simulink model "simple_controll"  (R2015b)
settings: Solver=FixedStepAuto  StartTime=0  StopTime=10  FixedStep=10*(1e-4)  RelTol=1e-3
undefined symbols (not defined in the file or in its folder): qc
libraries: simulink x4
settings Model: Creator=acsl  LastModifiedBy=acsl

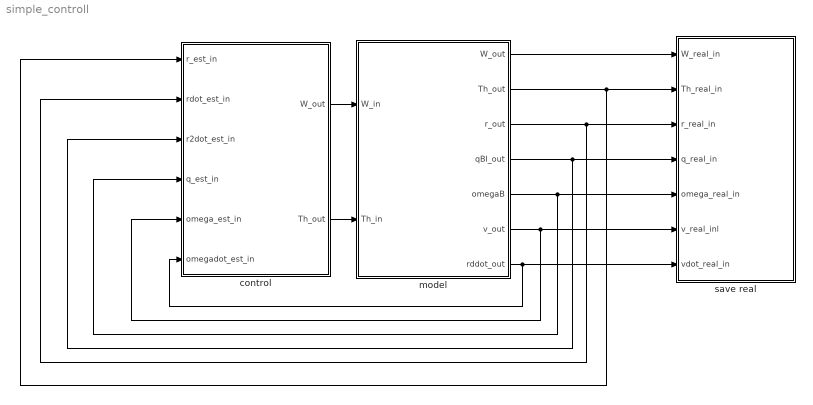
== system simple_controll ==
  control : Subsystem  InitFcn=init
  model : Subsystem
  save real : Subsystem
  wires:
  control/1(W_out) -> model/1(W_in)
  control/2(Th_out) -> model/2(Th_in)
  model/1(W_out) -> save real/1(W_real_in)
  model/2(Th_out) -> save real/2(Th_real_in), control/1(r_est_in)
  model/5(omegaB) -> save real/5(omega_real_in), control/4(q_est_in)
  model/6(v_out) -> save real/6(v_real_inl), control/5(omega_est_in)
  model/7(rddot_out) -> control/6(omegadot_est_in), save real/7(vdot_real_in)
  model/3(r_out) -> control/2(rdot_est_in), save real/3(r_real_in)
  model/4(qBI_out) -> save real/4(q_real_in), control/3(r2dot_est_in)

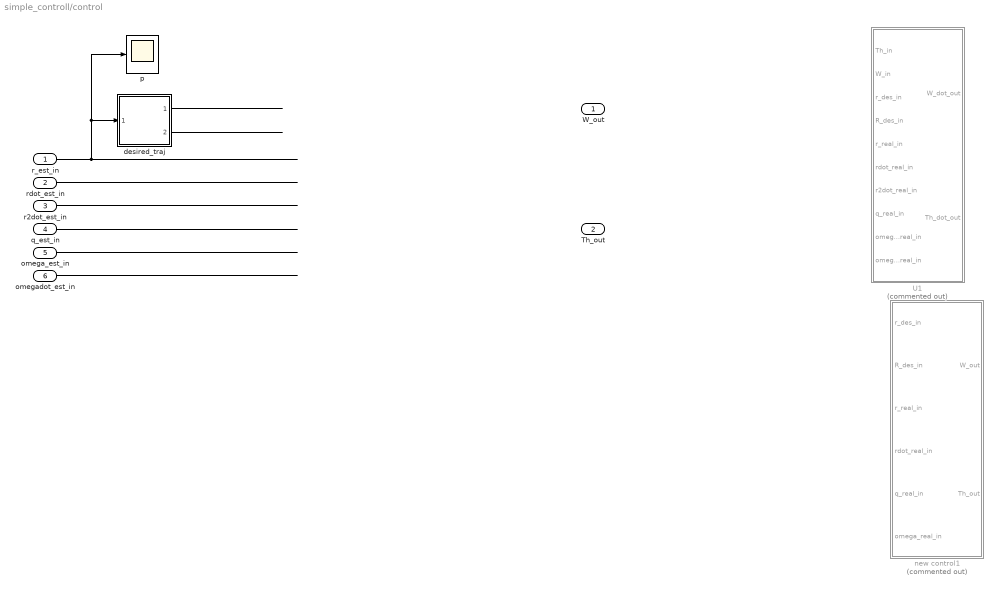
== system simple_controll/control ==
  r_est_in : Inport
  rdot_est_in : Inport  Port=2
  r2dot_est_in : Inport  Port=3
  q_est_in : Inport  Port=4
  omega_est_in : Inport  Port=5
  omegadot_est_in : Inport  Port=6
  U1 : Subsystem  Commented=on
  desired_traj : Subsystem
  new control1 : Subsystem  Commented=on
  p : Scope
  W_out : Outport
  Th_out : Outport  Port=2
  wires:
  desired_traj/1(r_des_out) -> ?
  desired_traj/2(R_des_out) -> ?
  omega_est_in/1 -> ?
  r2dot_est_in/1 -> ?
  q_est_in/1 -> ?
  rdot_est_in/1 -> ?
  r_est_in/1 -> desired_traj/1(r_real_in), p/1
  omegadot_est_in/1 -> ?

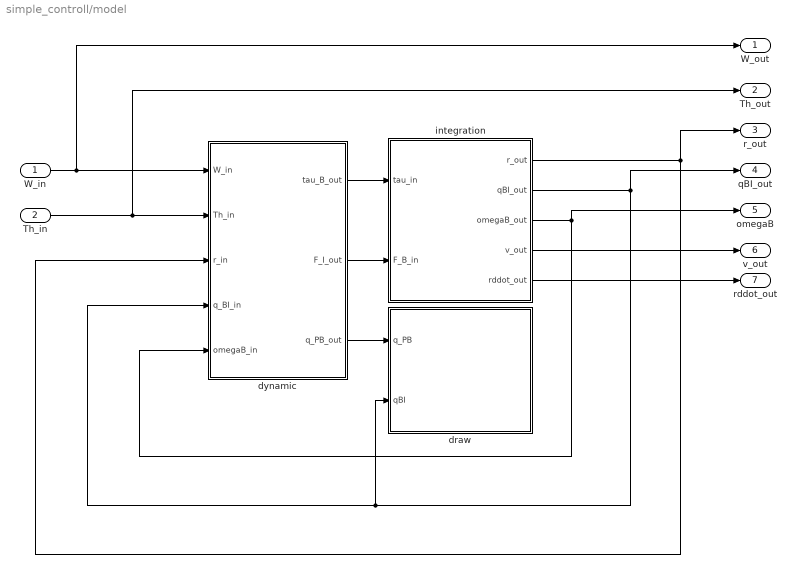
== system simple_controll/model ==
  W_in : Inport
  Th_in : Inport  Port=2
  draw : Subsystem
  dynamic : Subsystem  StopFcn=close all
  integration : Subsystem
  W_out : Outport
  Th_out : Outport  Port=2
  r_out : Outport  Port=3
  qBI_out : Outport  Port=4
  omegaB : Outport  Port=5
  v_out : Outport  Port=6
  rddot_out : Outport  Port=7
  wires:
  integration/1(r_out) -> dynamic/3(r_in), r_out/1
  dynamic/2(F_I_out) -> integration/2(F_B_in)
  integration/2(qBI_out) -> dynamic/4(q_BI_in), draw/2(qBI), qBI_out/1
  W_in/1 -> W_out/1, dynamic/1(W_in)
  dynamic/1(tau_B_out) -> integration/1(tau_in)
  integration/3(omegaB_out) -> dynamic/5(omegaB_in), omegaB/1
  Th_in/1 -> dynamic/2(Th_in), Th_out/1
  dynamic/3(q_PB_out) -> draw/1(q_PB)
  integration/5(rddot_out) -> rddot_out/1
  integration/4(v_out) -> v_out/1

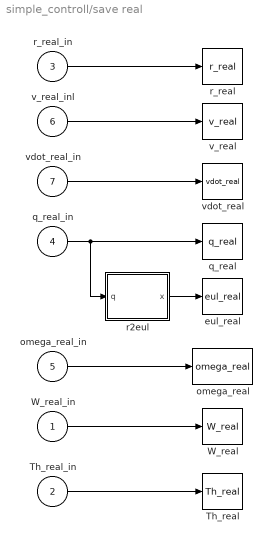
== system simple_controll/save real ==
  W_real_in : Inport
  Th_real_in : Inport  Port=2
  r_real_in : Inport  Port=3
  q_real_in : Inport  Port=4
  omega_real_in : Inport  Port=5
  v_real_inl : Inport  Port=6
  vdot_real_in : Inport  Port=7
  Th_real : ToWorkspace  VariableName=Th_real  SaveFormat=Timeseries  SampleTime=-1
  W_real : ToWorkspace  VariableName=W_real  SaveFormat=Timeseries  SampleTime=-1
  eul_real : ToWorkspace  VariableName=eul_real  SaveFormat=Timeseries  SampleTime=-1
  omega_real : ToWorkspace  VariableName=omega_real  SaveFormat=Timeseries  SampleTime=-1
  q_real : ToWorkspace  VariableName=q_real  SaveFormat=Timeseries  SampleTime=-1
  r2eul : MATLAB Function  TreatAsAtomicUnit=on
  r_real : ToWorkspace  VariableName=r_real  SaveFormat=Timeseries  SampleTime=-1
  v_real : ToWorkspace  VariableName=v_real  SaveFormat=Timeseries  SampleTime=-1
  vdot_real : ToWorkspace  VariableName=vdot_real  SaveFormat=Timeseries  SampleTime=-1
  wires:
  q_real_in/1 -> q_real/1, r2eul/1(q)
  r_real_in/1 -> r_real/1
  v_real_inl/1 -> v_real/1
  vdot_real_in/1 -> vdot_real/1
  r2eul/1(x) -> eul_real/1
  omega_real_in/1 -> omega_real/1
  Th_real_in/1 -> Th_real/1
  W_real_in/1 -> W_real/1

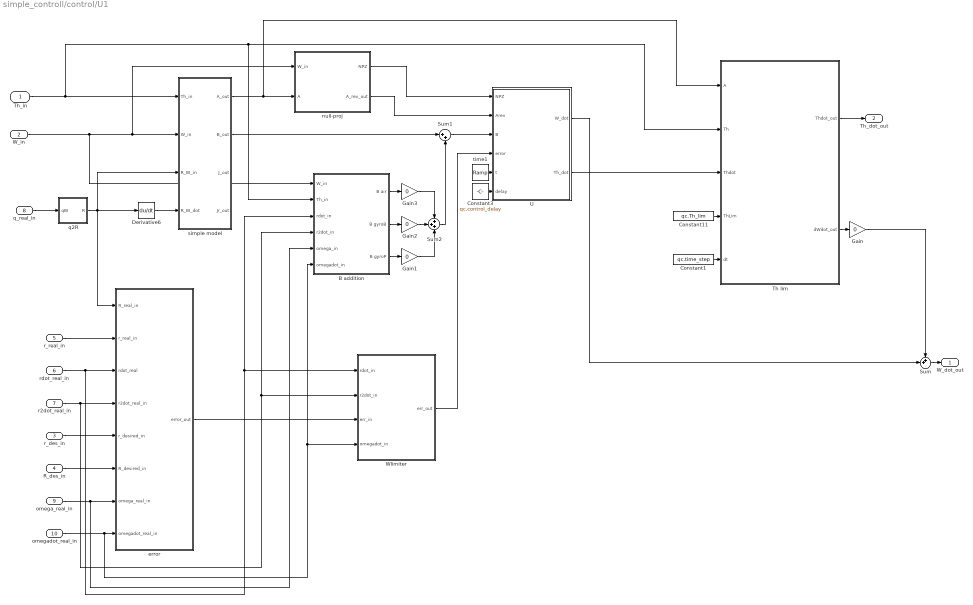
== system simple_controll/control/U1 ==
  Th_in : Inport
  W_in : Inport  Port=2
  r_des_in : Inport  Port=3
  R_des_in : Inport  Port=4
  r_real_in : Inport  Port=5
  rdot_real_in : Inport  Port=6
  r2dot_real_in : Inport  Port=7
  q_real_in : Inport  Port=8
  omega_real_in : Inport  Port=9
  omegadot_real_in : Inport  Port=10
  B addition : Subsystem
  Constant1 : Constant  Value=qc.time_step
  Constant11 : Constant  Value=qc.Th_lim
  Constant3 : Constant  Value=qc.control_delay
  Derivative6 : Derivative
  Gain{,1..3} (4 alike) : Gain  Gain=0
  Sum : Sum  Inputs=++|
  Sum1 : Sum  Inputs=|++
  Sum2 : Sum  Inputs=+++
  Th lim : MATLAB Function  TreatAsAtomicUnit=on
  U : MATLAB Function  TreatAsAtomicUnit=on
  Wlimiter : Subsystem
  error : Subsystem
  null-proj : Subsystem
  q2R : MATLAB Function  TreatAsAtomicUnit=on
  simple model : Subsystem
  time1 : simulink/Sources/Ramp  slope=1  start=0  X0=0
  W_dot_out : Outport
  Th_dot_out : Outport  Port=2
  wires:
  q_real_in/1 -> q2R/1(qBI)
  time1/1 -> U/5(t)
  null-proj/1(NPZ) -> U/1(NPZ)
  Constant3/1 -> U/6(delay)
  q2R/1(R) -> simple model/3(R_BI_in), error/1(R_real_in), Derivative6/1
  Th_in/1 -> B addition/2(Th_in), Th lim/2(Th), simple model/1(Th_in)
  Derivative6/1 -> simple model/4(R_BI_dot)
  simple model/1(A_out) -> Th lim/1(A), null-proj/2(A)
  r_real_in/1 -> error/2(r_real_in)
  r_des_in/1 -> error/5(r_desired_in)
  R_des_in/1 -> error/6(R_desired_in)
  W_in/1 -> B addition/1(W_in), simple model/2(W_in), null-proj/1(W_in)
  null-proj/2(A_rev_out) -> U/2(Arev)
  omega_real_in/1 -> error/7(omega_real_in), B addition/5(omega_in)
  rdot_real_in/1 -> error/3(rdot_real), Wlimiter/1(rdot_in), B addition/3(rdot_in)
  r2dot_real_in/1 -> error/4(r2dot_real_in), Wlimiter/2(r2dot_in), B addition/4(r2dot_in)
  omegadot_real_in/1 -> error/8(omegadot_real_in), Wlimiter/4(omegadot_in), B addition/6(omegadot_in)
  Constant11/1 -> Th lim/4(ThLim)
  U/1(W_dot) -> Sum/2
  Sum/1 -> W_dot_out/1
  Th lim/2(dWdot_out) -> Gain/1
  Constant1/1 -> Th lim/5(dt)
  U/2(Th_dot) -> Th lim/3(Thdot)
  Gain/1 -> Sum/1
  Th lim/1(Thdot_out) -> Th_dot_out/1
  simple model/2(B_out) -> Sum1/1
  Sum1/1 -> U/3(B)
  B addition/2(B gyroB) -> Gain2/1
  B addition/1(B air) -> Gain3/1
  Sum2/1 -> Sum1/2
  B addition/3(B gyroP) -> Gain1/1
  Gain1/1 -> Sum2/3
  Gain2/1 -> Sum2/2
  Gain3/1 -> Sum2/1
  error/1(error_out) -> Wlimiter/3(err_in)
  Wlimiter/1(err_out) -> U/4(error)

== system simple_controll/control/desired_traj ==
  r_real_in : Inport
  To Workspace1 : ToWorkspace  VariableName=time  SaveFormat=Timeseries  SampleTime=-1
  To Workspace2 : ToWorkspace  VariableName=r_des  SaveFormat=Timeseries  SampleTime=-1
  To Workspace6 : ToWorkspace  VariableName=eul_des  SaveFormat=Timeseries  SampleTime=-1
  time : simulink/Sources/Ramp  slope=1  start=0  X0=0
  traj : MATLAB Function  TreatAsAtomicUnit=on
  r_des_out : Outport
  R_des_out : Outport  Port=2
  wires:
  traj/2(R_des) -> R_des_out/1
  time/1 -> To Workspace1/1, traj/1(t)
  traj/3(eul_des) -> To Workspace6/1
  r_real_in/1 -> traj/2(rr)
  traj/1(r_des) -> To Workspace2/1, r_des_out/1

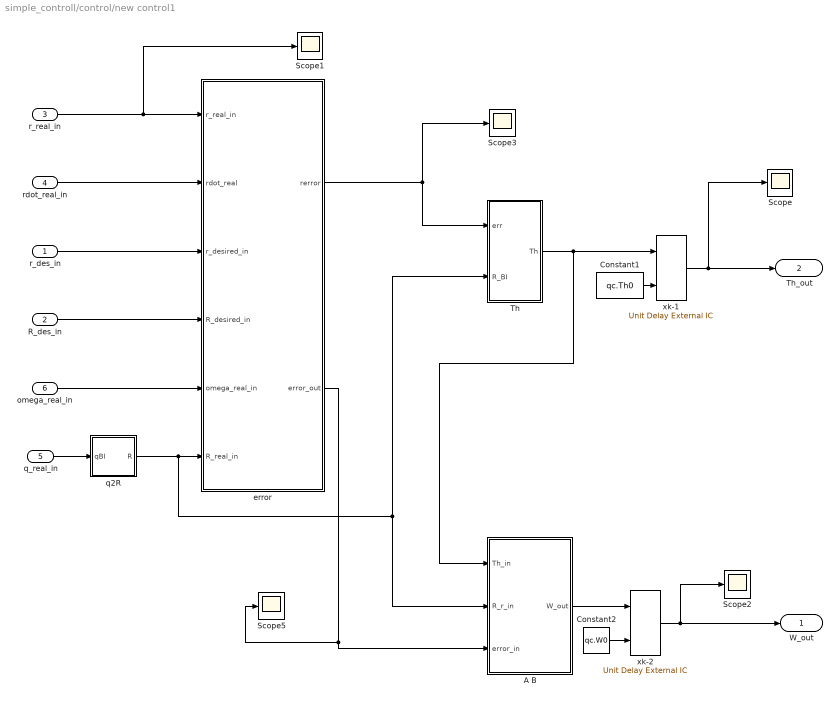
== system simple_controll/control/new control1 ==
  r_des_in : Inport
  R_des_in : Inport  Port=2
  r_real_in : Inport  Port=3
  rdot_real_in : Inport  Port=4
  q_real_in : Inport  Port=5
  omega_real_in : Inport  Port=6
  A B : Subsystem
  Constant1 : Constant  Value=qc.Th0
  Constant2 : Constant  Value=qc.W0
  Scope{,1..3,5} (5 alike) : Scope
  Th : MATLAB Function  TreatAsAtomicUnit=on
  error : Subsystem
  q2R : MATLAB Function  TreatAsAtomicUnit=on
  xk-1 : simulink/Additional Math & Discrete/Additional Discrete/Unit Delay External IC  tsamp=-1
  xk-2 : simulink/Additional Math & Discrete/Additional Discrete/Unit Delay External IC  tsamp=-1
  W_out : Outport
  Th_out : Outport  Port=2
  wires:
  Th/1(Th) -> xk-1/1, A B/1(Th_in)
  xk-1/1 -> Scope/1, Th_out/1
  error/1(rerror) -> Scope3/1, Th/1(err)
  error/2(error_out) -> Scope5/1, A B/3(error_in)
  A B/1(W_out) -> xk-2/1
  xk-2/1 -> W_out/1, Scope2/1
  Constant2/1 -> xk-2/2
  Constant1/1 -> xk-1/2
  q2R/1(R) -> error/6(R_real_in), A B/2(R_r_in), Th/2(R_BI)
  rdot_real_in/1 -> error/2(rdot_real)
  omega_real_in/1 -> error/5(omega_real_in)
  R_des_in/1 -> error/4(R_desired_in)
  r_des_in/1 -> error/3(r_desired_in)
  r_real_in/1 -> error/1(r_real_in), Scope1/1
  q_real_in/1 -> q2R/1(qBI)

== system simple_controll/model/draw ==
  q_PB : Inport
  qBI : Inport  Port=2
  Constant : Constant  Value=qc.rays
  Constant1 : Constant  Value=qc.l
  Constant2 : Constant  Value=qc.draw_on
  Rate Transition : RateTransition
  Rate Transition1 : RateTransition
  draw : MATLAB Function  TreatAsAtomicUnit=on  SystemSampleTime=qc.draw_tick
  wires:
  Constant1/1 -> draw/4(l)
  q_PB/1 -> Rate Transition1/1
  Rate Transition1/1 -> draw/2(q_PB)
  Constant/1 -> draw/3(rays)
  Rate Transition/1 -> draw/1(q_BI)
  qBI/1 -> Rate Transition/1
  Constant2/1 -> draw/5(draw_on)

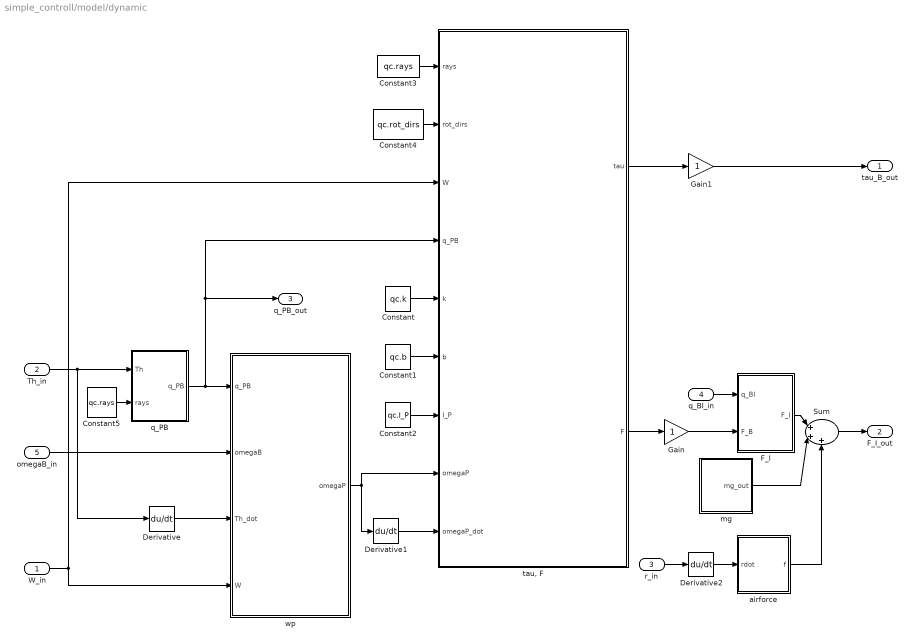
== system simple_controll/model/dynamic ==
  W_in : Inport
  Th_in : Inport  Port=2
  r_in : Inport  Port=3
  q_BI_in : Inport  Port=4
  omegaB_in : Inport  Port=5
  Constant : Constant  Value=qc.k
  Constant1 : Constant  Value=qc.b
  Constant2 : Constant  Value=qc.I_P
  Constant3 : Constant  Value=qc.rays
  Constant4 : Constant  Value=qc.rot_dirs
  Constant5 : Constant  Value=qc.rays
  Derivative : Derivative
  Derivative1 : Derivative
  Derivative2 : Derivative
  F_I : MATLAB Function  TreatAsAtomicUnit=on
  Gain : Gain
  Gain1 : Gain
  Sum : Sum  Inputs=|+++
  airforce : Subsystem
  mg : Subsystem
  q_PB : MATLAB Function  TreatAsAtomicUnit=on
  "tau, F" : MATLAB Function  TreatAsAtomicUnit=on
  wp : MATLAB Function  TreatAsAtomicUnit=on
  tau_B_out : Outport
  F_I_out : Outport  Port=2
  q_PB_out : Outport  Port=3
  wires:
  Th_in/1 -> q_PB/1(Th), Derivative/1
  q_PB/1(q_PB) -> "tau, F"/4(q_PB), q_PB_out/1, wp/1(q_PB)
  omegaB_in/1 -> wp/2(omegaB)
  Derivative/1 -> wp/3(Th_dot)
  W_in/1 -> "tau, F"/3(W), wp/4(W)
  wp/1(omegaP) -> Derivative1/1, "tau, F"/8(omegaP)
  Constant/1 -> "tau, F"/5(k)
  Constant1/1 -> "tau, F"/6(b)
  Constant2/1 -> "tau, F"/7(I_P)
  "tau, F"/2(F) -> Gain/1
  Constant3/1 -> "tau, F"/1(rays)
  Constant4/1 -> "tau, F"/2(rot_dirs)
  Gain1/1 -> tau_B_out/1
  Constant5/1 -> q_PB/2(rays)
  q_BI_in/1 -> F_I/1(q_BI)
  Gain/1 -> F_I/2(F_B)
  F_I/1(F_I) -> Sum/1
  mg/1(mg_out) -> Sum/2
  Sum/1 -> F_I_out/1
  r_in/1 -> Derivative2/1
  airforce/1(f) -> Sum/3
  "tau, F"/1(tau) -> Gain1/1
  Derivative1/1 -> "tau, F"/9(omegaP_dot)
  Derivative2/1 -> airforce/1(rdot)

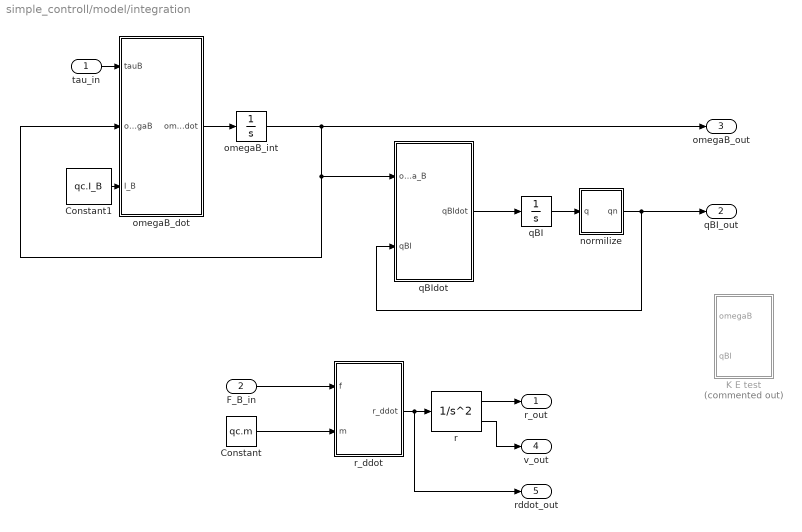
== system simple_controll/model/integration ==
  tau_in : Inport
  F_B_in : Inport  Port=2
  Constant : Constant  Value=qc.m
  Constant1 : Constant  Value=qc.I_B
  K E test : Subsystem  Commented=on
  normilize : MATLAB Function  TreatAsAtomicUnit=on
  omegaB_dot : MATLAB Function  TreatAsAtomicUnit=on
  omegaB_int : Integrator  InitialCondition=qc.omegaB0
  qBI : Integrator  InitialCondition=qc.qBI0
  qBIdot : MATLAB Function  TreatAsAtomicUnit=on
  r : SecondOrderIntegrator  ICX=qc.r0  ICDXDT=qc.v0
  r_ddot : MATLAB Function  TreatAsAtomicUnit=on
  r_out : Outport
  qBI_out : Outport  Port=2
  omegaB_out : Outport  Port=3
  v_out : Outport  Port=4
  rddot_out : Outport  Port=5
  wires:
  r/1 -> r_out/1
  r_ddot/1(r_ddot) -> rddot_out/1, r/1
  Constant/1 -> r_ddot/2(m)
  omegaB_int/1 -> omegaB_out/1, qBIdot/1(omega_B), omegaB_dot/2(omegaB)
  Constant1/1 -> omegaB_dot/3(I_B)
  tau_in/1 -> omegaB_dot/1(tauB)
  qBIdot/1(qBIdot) -> qBI/1
  qBI/1 -> normilize/1(q)
  normilize/1(qn) -> qBI_out/1, qBIdot/2(qBI)
  F_B_in/1 -> r_ddot/1(f)
  omegaB_dot/1(omegaB_dot) -> omegaB_int/1
  r/2 -> v_out/1

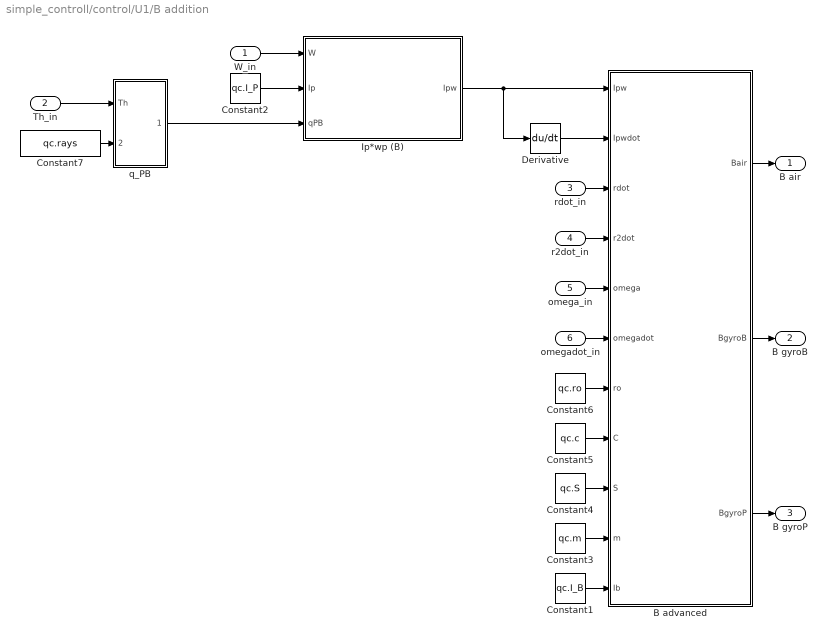
== system simple_controll/control/U1/B addition ==
  W_in : Inport
  Th_in : Inport  Port=2
  rdot_in : Inport  Port=3
  r2dot_in : Inport  Port=4
  omega_in : Inport  Port=5
  omegadot_in : Inport  Port=6
  B advanced : MATLAB Function  TreatAsAtomicUnit=on
  Constant1 : Constant  Value=qc.I_B
  Constant2 : Constant  Value=qc.I_P
  Constant3 : Constant  Value=qc.m
  Constant4 : Constant  Value=qc.S
  Constant5 : Constant  Value=qc.c
  Constant6 : Constant  Value=qc.ro
  Constant7 : Constant  Value=qc.rays
  Derivative : Derivative
  Ip*wp (B) : MATLAB Function  TreatAsAtomicUnit=on
  q_PB : MATLAB Function  TreatAsAtomicUnit=on
  B air : Outport
  B gyroB : Outport  Port=2
  B gyroP : Outport  Port=3
  wires:
  Constant4/1 -> B advanced/9(S)
  Constant3/1 -> B advanced/10(m)
  rdot_in/1 -> B advanced/3(rdot)
  Constant5/1 -> B advanced/8(C)
  B advanced/1(Bair) -> B air/1
  omegadot_in/1 -> B advanced/6(omegadot)
  B advanced/3(BgyroP) -> B gyroP/1
  omega_in/1 -> B advanced/5(omega)
  B advanced/2(BgyroB) -> B gyroB/1
  r2dot_in/1 -> B advanced/4(r2dot)
  Constant6/1 -> B advanced/7(ro)
  Constant2/1 -> Ip*wp (B)/2(Ip)
  Constant1/1 -> B advanced/11(Ib)
  Th_in/1 -> q_PB/1(Th)
  Constant7/1 -> q_PB/2(rays)
  Derivative/1 -> B advanced/2(Ipwdot)
  Ip*wp (B)/1(Ipw) -> Derivative/1, B advanced/1(Ipw)
  W_in/1 -> Ip*wp (B)/1(W)
  q_PB/1(q_PB) -> Ip*wp (B)/3(qPB)

== system simple_controll/control/U1/Wlimiter ==
  rdot_in : Inport
  r2dot_in : Inport  Port=2
  err_in : Inport  Port=3
  omegadot_in : Inport  Port=4
  Constant10 : Constant  Value=qc.m
  Constant5 : Constant  Value=qc.r2dot_control_signal_lim
  Constant6 : Constant  Value=qc.time_step
  Constant7 : Constant  Value=qc.g
  Constant8 : Constant  Value=qc.wdot_control_signal_lim
  W lim : MATLAB Function  TreatAsAtomicUnit=on
  airforce : Subsystem
  err_out : Outport
  wires:
  W lim/1(err_out) -> err_out/1
  r2dot_in/1 -> W lim/2(r2dot)
  rdot_in/1 -> airforce/1(rdot)
  omegadot_in/1 -> W lim/3(wdot)
  err_in/1 -> W lim/4(err_in)
  Constant5/1 -> W lim/5(rlim)
  Constant6/1 -> W lim/7(tick)
  Constant7/1 -> W lim/8(g)
  Constant8/1 -> W lim/6(wlim)
  airforce/1(f) -> W lim/1(airforce)
  Constant10/1 -> W lim/9(m)

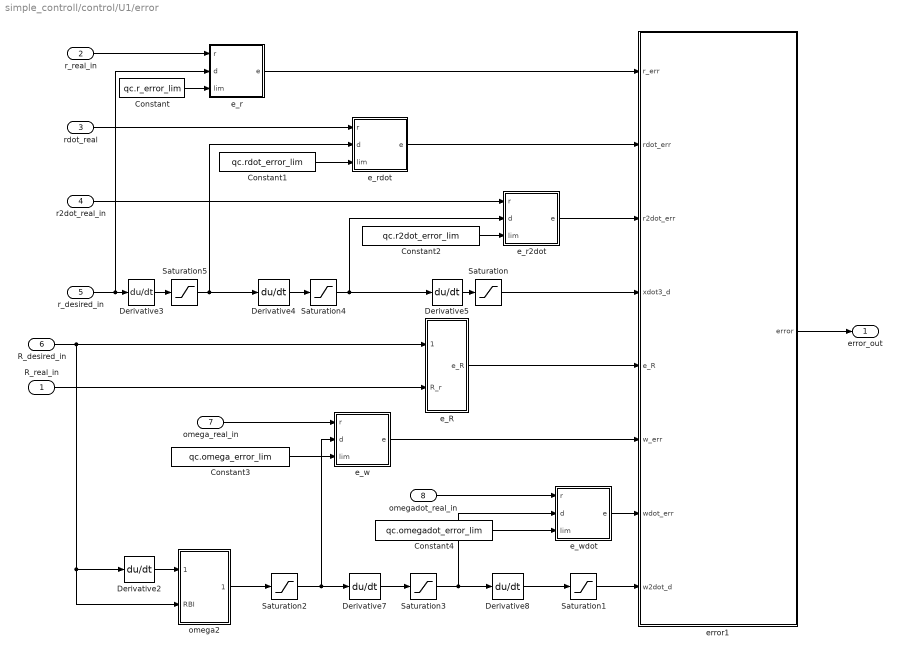
== system simple_controll/control/U1/error ==
  R_real_in : Inport
  r_real_in : Inport  Port=2
  rdot_real : Inport  Port=3
  r2dot_real_in : Inport  Port=4
  r_desired_in : Inport  Port=5
  R_desired_in : Inport  Port=6
  omega_real_in : Inport  Port=7
  omegadot_real_in : Inport  Port=8
  Constant : Constant  Value=qc.r_error_lim
  Constant1 : Constant  Value=qc.rdot_error_lim
  Constant2 : Constant  Value=qc.r2dot_error_lim
  Constant3 : Constant  Value=qc.omega_error_lim
  Constant4 : Constant  Value=qc.omegadot_error_lim
  Derivative{2..5,7..8} (6 alike) : Derivative
  Saturation : Saturate  UpperLimit=qc.r2dot_des_lim  LowerLimit=-qc.r2dot_des_lim
  Saturation1 : Saturate  UpperLimit=qc.w_des_lim/4  LowerLimit=-qc.w_des_lim/4
  Saturation2 : Saturate  UpperLimit=qc.w_des_lim  LowerLimit=-qc.w_des_lim
  Saturation3 : Saturate  UpperLimit=qc.w_des_lim/2  LowerLimit=-qc.w_des_lim/2
  Saturation4 : Saturate  UpperLimit=qc.r2dot_des_lim  LowerLimit=-qc.r2dot_des_lim
  Saturation5 : Saturate  UpperLimit=qc.rdot_des_lim  LowerLimit=-qc.rdot_des_lim
  e_R : MATLAB Function  TreatAsAtomicUnit=on
  e_r : MATLAB Function  TreatAsAtomicUnit=on
  e_r2dot : MATLAB Function  TreatAsAtomicUnit=on
  e_rdot : MATLAB Function  TreatAsAtomicUnit=on
  e_w : MATLAB Function  TreatAsAtomicUnit=on
  e_wdot : MATLAB Function  TreatAsAtomicUnit=on
  error1 : MATLAB Function  TreatAsAtomicUnit=on
  omega2 : MATLAB Function  TreatAsAtomicUnit=on
  error_out : Outport
  wires:
  R_real_in/1 -> e_R/2(R_r)
  Derivative2/1 -> omega2/1(RBIdot)
  R_desired_in/1 -> omega2/2(RBI), Derivative2/1, e_R/1(R_d)
  omega2/1(omega) -> Saturation2/1
  Derivative3/1 -> Saturation5/1
  Derivative7/1 -> Saturation3/1
  e_R/1(e_R) -> error1/5(e_R)
  Derivative4/1 -> Saturation4/1
  e_r/1(e) -> error1/1(r_err)
  Constant/1 -> e_r/3(lim)
  e_rdot/1(e) -> error1/2(rdot_err)
  rdot_real/1 -> e_rdot/1(r)
  r2dot_real_in/1 -> e_r2dot/1(r)
  e_r2dot/1(e) -> error1/3(r2dot_err)
  Derivative5/1 -> Saturation/1
  Constant1/1 -> e_rdot/3(lim)
  Constant2/1 -> e_r2dot/3(lim)
  e_w/1(e) -> error1/6(w_err)
  omega_real_in/1 -> e_w/1(r)
  Derivative8/1 -> Saturation1/1
  e_wdot/1(e) -> error1/7(wdot_err)
  omegadot_real_in/1 -> e_wdot/1(r)
  Constant3/1 -> e_w/3(lim)
  Constant4/1 -> e_wdot/3(lim)
  r_real_in/1 -> e_r/1(r)
  Saturation/1 -> error1/4(xdot3_d)
  Saturation1/1 -> error1/8(w2dot_d)
  r_desired_in/1 -> Derivative3/1, e_r/2(d)
  Saturation2/1 -> e_w/2(d), Derivative7/1
  Saturation3/1 -> Derivative8/1, e_wdot/2(d)
  Saturation4/1 -> e_r2dot/2(d), Derivative5/1
  Saturation5/1 -> e_rdot/2(d), Derivative4/1
  error1/1(error) -> error_out/1

== system simple_controll/control/U1/null-proj ==
  W_in : Inport
  A : Inport  Port=2
  Arev : MATLAB Function  TreatAsAtomicUnit=on
  Constant1 : Constant  Value=qc.wnorm
  Constant2 : Constant  Value=qc.wmin
  Np*Z : MATLAB Function  TreatAsAtomicUnit=on
  NPZ : Outport
  A_rev_out : Outport  Port=2
  wires:
  Arev/1(Arev) -> A_rev_out/1, Np*Z/2(Arev)
  W_in/1 -> Np*Z/3(W)
  Constant1/1 -> Np*Z/5(Wnorm)
  Constant2/1 -> Np*Z/4(Wmin)
  Np*Z/1(NPZ) -> NPZ/1
  A/1 -> Np*Z/1(A), Arev/1(A)

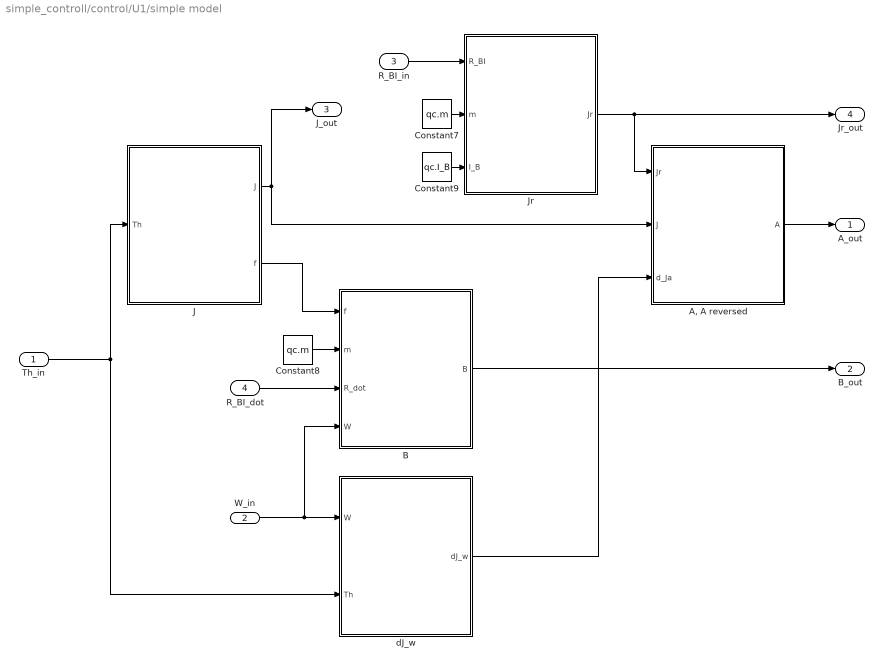
== system simple_controll/control/U1/simple model ==
  Th_in : Inport
  W_in : Inport  Port=2
  R_BI_in : Inport  Port=3
  R_BI_dot : Inport  Port=4
  "A, A reversed" : MATLAB Function  TreatAsAtomicUnit=on
  B : MATLAB Function  TreatAsAtomicUnit=on
  Constant7 : Constant  Value=qc.m
  Constant8 : Constant  Value=qc.m
  Constant9 : Constant  Value=qc.I_B
  J : MATLAB Function  TreatAsAtomicUnit=on
  Jr : MATLAB Function  TreatAsAtomicUnit=on
  dJ_w : MATLAB Function  TreatAsAtomicUnit=on
  A_out : Outport
  B_out : Outport  Port=2
  J_out : Outport  Port=3
  Jr_out : Outport  Port=4
  wires:
  Constant9/1 -> Jr/3(I_B)
  Th_in/1 -> J/1(Th), dJ_w/2(Th)
  dJ_w/1(dJ_w) -> "A, A reversed"/3(d_Ja)
  Constant7/1 -> Jr/2(m)
  Constant8/1 -> B/2(m)
  J/2(f) -> B/1(f)
  J/1(J) -> J_out/1, "A, A reversed"/2(J)
  B/1(B) -> B_out/1
  "A, A reversed"/1(A) -> A_out/1
  R_BI_dot/1 -> B/3(R_dot)
  R_BI_in/1 -> Jr/1(R_BI)
  W_in/1 -> B/4(W), dJ_w/1(W)
  Jr/1(Jr) -> "A, A reversed"/1(Jr), Jr_out/1

== system simple_controll/control/new control1/A B ==
  Th_in : Inport
  R_r_in : Inport  Port=2
  error_in : Inport  Port=3
  "A, Apinv " : MATLAB Function  TreatAsAtomicUnit=on
  Constant1 : Constant  Value=qc.g
  Constant7 : Constant  Value=qc.m
  Constant9 : Constant  Value=qc.I_B
  J : MATLAB Function  TreatAsAtomicUnit=on
  Jr : MATLAB Function  TreatAsAtomicUnit=on
  U(W) : MATLAB Function  TreatAsAtomicUnit=on
  W_out : Outport
  wires:
  U(W)/1(W) -> W_out/1
  error_in/1 -> U(W)/3(error)
  "A, Apinv "/2(Apinv) -> U(W)/2(pinvA)
  Constant1/1 -> U(W)/1(g)
  J/1(J) -> "A, Apinv "/1(J)
  Jr/1(Jr) -> "A, Apinv "/2(Jr)
  R_r_in/1 -> Jr/1(R_BI)
  Constant9/1 -> Jr/3(I_B)
  Constant7/1 -> Jr/2(m)
  Th_in/1 -> J/1(Th)

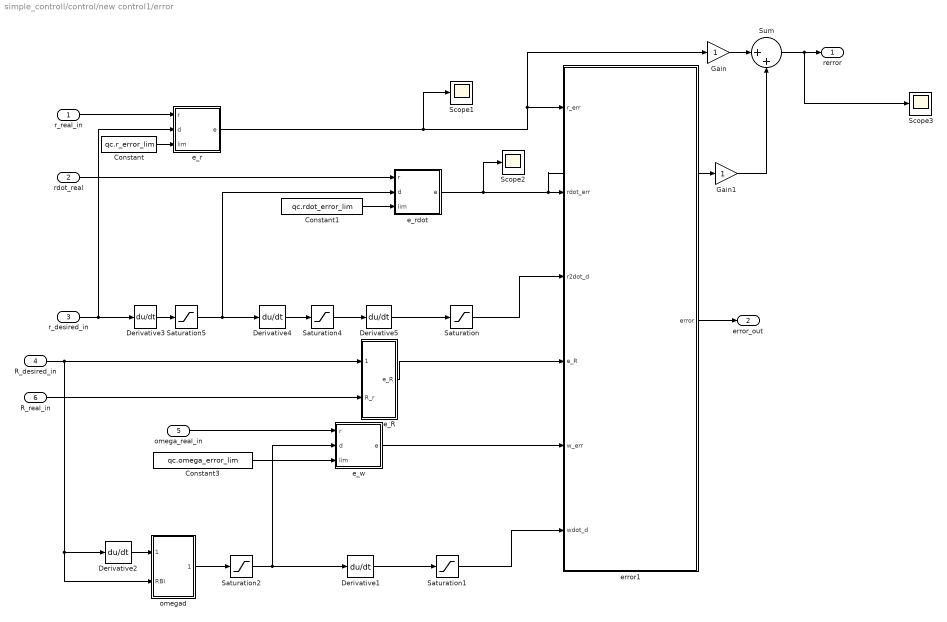
== system simple_controll/control/new control1/error ==
  r_real_in : Inport
  rdot_real : Inport  Port=2
  r_desired_in : Inport  Port=3
  R_desired_in : Inport  Port=4
  omega_real_in : Inport  Port=5
  R_real_in : Inport  Port=6
  Constant : Constant  Value=qc.r_error_lim
  Constant1 : Constant  Value=qc.rdot_error_lim
  Constant3 : Constant  Value=qc.omega_error_lim
  Derivative{1..5} (5 alike) : Derivative
  Gain : Gain
  Gain1 : Gain
  Saturation : Saturate  UpperLimit=qc.r2dot_des_lim  LowerLimit=-qc.r2dot_des_lim
  Saturation1 : Saturate  UpperLimit=qc.w_des_lim/2  LowerLimit=-qc.w_des_lim/2
  Saturation2 : Saturate  UpperLimit=qc.w_des_lim  LowerLimit=-qc.w_des_lim
  Saturation4 : Saturate  UpperLimit=qc.r2dot_des_lim  LowerLimit=-qc.r2dot_des_lim
  Saturation5 : Saturate  UpperLimit=qc.rdot_des_lim  LowerLimit=-qc.rdot_des_lim
  Scope1 : Scope
  Scope2 : Scope
  Scope3 : Scope
  Sum : Sum  Inputs=|++
  e_R : MATLAB Function  TreatAsAtomicUnit=on
  e_r : MATLAB Function  TreatAsAtomicUnit=on
  e_rdot : MATLAB Function  TreatAsAtomicUnit=on
  e_w : MATLAB Function  TreatAsAtomicUnit=on
  error1 : MATLAB Function  TreatAsAtomicUnit=on
  omegad : MATLAB Function  TreatAsAtomicUnit=on
  rerror : Outport
  error_out : Outport  Port=2
  wires:
  Gain1/1 -> Sum/2
  Gain/1 -> Sum/1
  Sum/1 -> rerror/1, Scope3/1
  Saturation1/1 -> error1/6(wdot_d)
  Derivative1/1 -> Saturation1/1
  Saturation/1 -> error1/3(r2dot_d)
  R_real_in/1 -> e_R/2(R_r)
  error1/1(error) -> error_out/1
  Saturation5/1 -> Derivative4/1, e_rdot/2(d)
  Saturation4/1 -> Derivative5/1
  Saturation2/1 -> e_w/2(d), Derivative1/1
  r_desired_in/1 -> e_r/2(d), Derivative3/1
  r_real_in/1 -> e_r/1(r)
  Constant3/1 -> e_w/3(lim)
  omega_real_in/1 -> e_w/1(r)
  e_w/1(e) -> error1/5(w_err)
  Constant1/1 -> e_rdot/3(lim)
  Derivative5/1 -> Saturation/1
  rdot_real/1 -> e_rdot/1(r)
  e_rdot/1(e) -> error1/2(rdot_err), Gain1/1, Scope2/1
  Constant/1 -> e_r/3(lim)
  e_r/1(e) -> error1/1(r_err), Gain/1, Scope1/1
  Derivative4/1 -> Saturation4/1
  e_R/1(e_R) -> error1/4(e_R)
  Derivative3/1 -> Saturation5/1
  omegad/1(omega) -> Saturation2/1
  R_desired_in/1 -> e_R/1(R_d), Derivative2/1, omegad/2(RBI)
  Derivative2/1 -> omegad/1(RBIdot)

== system simple_controll/model/dynamic/airforce ==
  rdot : Inport
  Constant10 : Constant  Value=qc.S
  Constant8 : Constant  Value=qc.ro
  Constant9 : Constant  Value=qc.c
  air force I : MATLAB Function  TreatAsAtomicUnit=on
  f : Outport
  wires:
  air force I/1(f) -> f/1
  Constant9/1 -> air force I/3(c)
  Constant10/1 -> air force I/4(S)
  Constant8/1 -> air force I/2(ro)
  rdot/1 -> air force I/1(r_dot)

== system simple_controll/model/dynamic/mg ==
  Constant6 : Constant  Value=qc.m
  Constant7 : Constant  Value=qc.g
  mg : MATLAB Function  TreatAsAtomicUnit=on
  mg_out : Outport
  wires:
  Constant7/1 -> mg/2(g)
  Constant6/1 -> mg/1(m)
  mg/1(mg) -> mg_out/1

== system simple_controll/model/integration/K E test ==
  omegaB : Inport
  qBI : Inport  Port=2
  Constant2 : Constant  Value=qc.I_B
  "K, E" : MATLAB Function  TreatAsAtomicUnit=on
  rgb : Scope
  rgb1 : Scope
  wires:
  omegaB/1 -> "K, E"/2(omega_B)
  qBI/1 -> "K, E"/3(qBI)
  "K, E"/1(K) -> rgb/1
  "K, E"/2(E) -> rgb1/1
  Constant2/1 -> "K, E"/1(I_B)

== system simple_controll/control/U1/Wlimiter/airforce ==
  rdot : Inport
  Constant10 : Constant  Value=qc.S
  Constant8 : Constant  Value=qc.ro
  Constant9 : Constant  Value=qc.c
  air force I : MATLAB Function  TreatAsAtomicUnit=on
  f : Outport
  wires:
  air force I/1(f) -> f/1
  Constant9/1 -> air force I/3(c)
  Constant10/1 -> air force I/4(S)
  Constant8/1 -> air force I/2(ro)
  rdot/1 -> air force I/1(r_dot)

== matlab function simple_controll/model/dynamic/wp ==
  data: q_PB input; omegaP output; omegaB input; Th_dot input; W input
function omegaP  = fcn(q_PB, omegaB, Th_dot, W)

omegaP = zeros(4*3,1);
for i = 1:4
    
    q_pb = q_PB(:, i);
    q_bp = quatDual(q_pb);
    w = sign(W(i))*sqrt(abs(W(i)));
    omegaP(3*i-2:3*i, 1) = quatRotate(q_bp, omegaB) + [Th_dot(i); 0; w];
    w1 = [0;0;w];
    th1 = [Th_dot(i); 0; 0];
    Ob1 = quatRotate(q_bp, omegaB);
end

== matlab function simple_controll/model/integration/normilize ==
  data: q input; qn output
function qn  = fcn(q)
qn = q / norm(q);

== matlab function simple_controll/model/dynamic/tau, F ==
  data: rays input; rot_dirs input; W input; q_PB input; k input; b input; I_P input; omegaP input; omegaP_dot input; tau output; F output
function [tau, F]= fcn(rays, rot_dirs, W, q_PB, k, b, I_P, omegaP, omegaP_dot)

tau = [0;0;0];
F = [0;0;0];
Jt2 = zeros(3, 4);
for i = 1:4
    ray = rays(3*i-2:3*i);
    dir = rot_dirs(i);
    omega_p = omegaP(3*i-2:3*i);
    omega_pz = omega_p(3);
    omega_p_dot = omegaP_dot(3*i-2:3*i);
    q_pb = q_PB(:, i);

    fp = dir*[0;0;k*W(i)];
    fb = quatRotate(q_pb,fp);
    
    tau_p_ext = [0;0;-b*abs(omega_pz)*omega_pz];
    tau_p = 1*I_P*omega_p_dot + 1*cross(omega_p, I_P*omega_p) - tau_p_ext;
    tau_b = cross(ray, fb) - quatRotate(q_pb, tau_p);
    
    tau = tau + tau_b;
    
    Jt2(:,i) = tau_b/W(i);
    
    F = F + fb;
end

== matlab function simple_controll/model/dynamic/mg/mg ==
  data: m input; mg output; g input
function mg  = fcn(m, g)
mg = m*g;

== matlab function simple_controll/model/integration/r_ddot ==
  data: r_ddot output; f input; m input
function r_ddot  = fcn(f, m)

r_ddot = f/m;

== matlab function simple_controll/save real/r2eul ==
  data: q input; x output
function x = fnc(q)
eul = quat2eul(q');
x = eul';
end

== matlab function simple_controll/model/integration/omegaB_dot ==
  data: tauB input; omegaB_dot output; omegaB input; I_B input
function omegaB_dot  = fcn(tauB, omegaB, I_B)
omegaB_dot = I_B^(-1) * (tauB - 1*cross(omegaB, I_B * omegaB));

== matlab function simple_controll/model/dynamic/F_I ==
  data: q_BI input; F_I output; F_B input
function F_I  = fcn(q_BI, F_B)
F_I = quatRotate(q_BI, F_B);

== matlab function simple_controll/model/integration/qBIdot ==
  data: omega_B input; qBIdot output; qBI input
function qBIdot  = fcn(omega_B, qBI)
qw = [0;omega_B];
qBIdot = 0.5*quatMultiply(qBI, qw);

== matlab function simple_controll/model/draw/draw ==
  data: q_BI input; q_PB input; rays input; l input; draw_on input
function drawFly(q_BI, q_PB, rays, l, draw_on)
drawFly(q_BI, q_PB, rays, l, draw_on)
end

== matlab function simple_controll/model/integration/K E test/K, E ==
  data: I_B input; omega_B input; qBI input; K output; E output
function [K, E] = fcn(I_B, omega_B, qBI)
K_B = I_B*omega_B;
K = quatRotate(qBI, K_B);
E = omega_B'*I_B*omega_B / 2;

== matlab function simple_controll/control/U1/B addition/B advanced ==
  data: Ipw input; Ipwdot input; rdot input; r2dot input; omega input; omegadot input; ro input; C input; S input; m input; Bair output; Ib input; BgyroB output; BgyroP output
function [Bair, BgyroB, BgyroP]  = fcn(Ipw, Ipwdot, rdot, r2dot, omega, omegadot, ro, C, S, m, Ib)
v = norm(rdot);
vdot = norm(r2dot);
Bair1 = -0.5*ro*C*S*(v*r2dot+vdot*rdot)/m;
Bair = [Bair1; zeros(3,1)];

BgyroB1 = (Ib^-1)*(cross(-omegadot, Ib*omega) + cross(-omega, Ib*omegadot));
BgyroB = [zeros(3,1); BgyroB1];

BgyroP = zeros(6, 1);
for i =1:4
    ipw = Ipw(:, i);
    ipwdot = Ipwdot(:, i);
    addition = (Ib^-1)*(cross(-omegadot, ipw) + cross(-omega, ipwdot));
    BgyroP = BgyroP + [zeros(3, 1); addition];
end

end

== matlab function simple_controll/control/U1/B addition/Ip*wp (B) ==
  data: W input; Ip input; qPB input; Ipw output
function Ipw   = fcn(W, Ip, qPB)

Ipw = zeros(3:4);
for i =1:4
    w = sign(W(i))*sqrt(abs(W(i)));
    qpb = qPB(:, i);
    omegaP = [0;0;w];
    Ipw(:,i) = Ip*omegaP;
    Ipw(:,i) = quatRotate(qpb, Ipw(:,i));
end

end

== matlab function simple_controll/control/desired_traj/traj ==
  data: r_des output; R_des output; t input; eul_des output; rr input
function [r_des, R_des, eul_des] = curve(t, rr)
[ r_des, R_des, eul_des ] = current_traj( t, rr);
end

== matlab function simple_controll/model/dynamic/q_PB ==
  data: Th input; q_PB output; rays input
function q_PB = fcn(Th, rays)
q_PB = quatPB(Th, rays);
end

== matlab function simple_controll/model/dynamic/airforce/air force I ==
  data: r_dot input; f output; ro input; c input; S input
function f = fcn(r_dot, ro, c, S)
f = -ro*c*S*norm(r_dot)*r_dot;

== matlab function simple_controll/control/U1/B addition/q_PB ==
  data: Th input; q_PB output; rays input
function q_PB = fcn(Th, rays)
ex = [1;0;0];
ez = [0;0;1];
q_PB = zeros(4, 4);
for i = 1:4
    ray = rays(3*i-2:3*i);
    cosAlpha = dot(ex, ray/norm(ray));
    alpha = acos(cosAlpha);
    if(ray(2) < 0)
        alpha = -alpha;
    end
    th = Th(i);
    qth = [cos(th/2);ex*sin(th/2)];
    qa = [cos(alpha/2);ez*sin(alpha/2)];
    q = quatMultiply(qa, qth);
    q_PB(:,i) = q;
end

== matlab function simple_controll/control/U1/Th lim ==
  data: A input; Th input; Thdot input; ThLim input; Thdot_out output; dWdot_out output; dt input
function [Thdot_out, dWdot_out]= fcn(A, Th, Thdot, ThLim, dt)

Thdot_out = Thdot;
dWdot_out = [0;0;0;0];

% k1 = abs((Th + 1*Th*dt) / ThLim);
% k2 = max(k1, 0);
% 
% d = -k1 .* Thdot;
% d = 1*d - 0*k2 .* (Th/dt);
% 
% Thdot_out = Thdot + d;
% Aw = A(:, 1:4);
% Ath = A(:, 5:8);
% AwP = pinv(Aw);
% dWdot_out = -AwP*Ath*d
end

== matlab function simple_controll/control/U1/U ==
  data: NPZ input; Arev input; B input; error input; W_dot output; Th_dot output; t input; delay input
function [W_dot, Th_dot]  = fcn(NPZ, Arev, B, error, t, delay)
U = zeros(8, 1);
if t > delay
    U = Arev*(error - B) + 1*NPZ;
end
W_dot = U(1:4);
Th_dot = U(5:8);
end

== matlab function simple_controll/control/U1/Wlimiter/W lim ==
  data: airforce input; r2dot input; wdot input; err_in input; err_out output; rlim input; wlim input; tick input; g input; m input
function err_out = fcn(airforce, r2dot, wdot, err_in, rlim, wlim, tick, g, m)

r3dot = err_in(1:3);
w2dot = err_in(4:6);


Fa = r2dot - g - airforce/m;

%% Zlim
% x = Fa .* [0;0;1];
% dx = r3dot*tick.* [0;0;1];
% r = Zlim;
% r3dotZ = find_dr(x, dx, r)/tick;
% 
% %% XY lim
% x = Fa .* [1;1;0];
% dx = r3dot*tick.* [1;1;0];
% r = XYlim;
% r3dotXY = find_dr(x, dx, r)/tick;


%% R ellipsoid lim
v = Fa;
dv = r3dot*tick;
c = rlim; a = c / sqrt(2); b = c / sqrt(2);
r3dot = find_dr_ellipsoid(v, dv, a, b, c)/tick;

%% Omega lim
% r3dot = r3dotXY + r3dotZ;
% 
% x = wdot;
% dx = w2dot*tick;
% r = wlim;
% w2dot = find_dr(x, dx, r)/tick;

%%
err_out = [r3dot; w2dot];
end

== matlab function simple_controll/control/U1/Wlimiter/airforce/air force I ==
  data: r_dot input; f output; ro input; c input; S input
function f = fcn(r_dot, ro, c, S)
f = -ro*c*S*norm(r_dot)*r_dot;

== matlab function simple_controll/control/U1/error/e_R ==
  data: R_d input; R_r input; e_R output size=3
function e_R = e_r(R_d, R_r)
Me_R = R_r'*R_d - R_d'*R_r;
e_R = 0.5*[-Me_R(2,3); Me_R(1,3); -Me_R(1,2)];
end

== matlab function simple_controll/control/U1/error/e_r ==
  data: r input; d input; e output size=3; lim input
function e = e_r(r, d, lim)
e = d - r;
n = norm(e);
if n < lim
    return;
end
e = lim*e/n;
end

== matlab function simple_controll/control/U1/error/e_r2dot ==
  data: r input; d input; e output size=3; lim input
function e = e_r(r, d, lim)
e = d - r;
n = norm(e);
if n < lim
    return;
end
e = lim*e/n;
end

== matlab function simple_controll/control/U1/error/e_rdot ==
  data: r input; d input; e output size=3; lim input
function e = e_r(r, d, lim)
e = d - r;
n = norm(e);
if n < lim
    return;
end
e = lim*e/n;
end

== matlab function simple_controll/control/U1/error/e_w ==
  data: r input; d input; e output size=3; lim input
function e = e_r(r, d, lim)
e = d - r;
n = norm(e);
if n < lim
    return;
end
e = lim*e/n;
end

== matlab function simple_controll/control/U1/error/e_wdot ==
  data: r input; d input; e output size=3; lim input
function e = e_r(r, d, lim)
e = d - r;
n = norm(e);
if n < lim
    return;
end
e = lim*e/n;
end

== matlab function simple_controll/control/U1/error/error1 ==
  data: r_err input; rdot_err input; error output; r2dot_err input; xdot3_d input; e_R input; w_err input; wdot_err input; w2dot_d input
function error = x_e(r_err, rdot_err, r2dot_err, xdot3_d, e_R, w_err, wdot_err, w2dot_d)
   
K2 = [1,0,0;
      0,1,0;
      0,0,1]*28.5;

K1 = [1,0,0;
      0,1,0;
      0,0,1]*271;

K0 =  [1,0,0;
       0,1,0;
       0,0,1]*857;
   
e_x = xdot3_d + K2*(r2dot_err) + K1*(rdot_err)+ K0*(r_err);

C2 =   [1,0,0;
        0,1,0;
        0,0,1]*45;

C1 =   [1,0,0;
        0,1,0;
        0,0,1]*675;

C0 =   [1,0,0;
        0,1,0;
        0,0,1.6]*3375;
          
e_r = w2dot_d + C2*(wdot_err) + C1*(w_err) + C0*(e_R);
e_r = 1*e_r*1;

error = [e_x; e_r];
end

== matlab function simple_controll/control/U1/error/omega2 ==
  data: omega output; RBIdot input; RBI input
function omega  = fcn(RBIdot, RBI)

R = RBI'*RBIdot;
omega = [-R(2,3); R(1,3); -R(1,2)];

== matlab function simple_controll/control/U1/null-proj/Arev ==
  data: A input; Arev output
function Arev    = fcn(A)
Arev = pinv(A);
end

== matlab function simple_controll/control/U1/null-proj/Np*Z ==
  data: A input; Arev input; NPZ output; W input; Wmin input; Wnorm input
function NPZ  = fcn(A, Arev, W, Wmin, Wnorm)

Z = zeros(8,1);

for i = 1:4
    Z(i) = sign(W(i))*calc_z(abs(W(i)), Wmin, Wnorm);
end

NPZ = (eye(8) - Arev*A) * Z;
end

== matlab function simple_controll/control/U1/q2R ==
  data: qBI input; R output
function R = q2R(qBI)
R = quat2matrix(qBI);
end

== matlab function simple_controll/control/U1/simple model/A, A reversed ==
  data: Jr input; J input; d_Ja input; A output
function A  = fcn(Jr, J, d_Ja)
A = Jr * [J d_Ja];
end

== matlab function simple_controll/control/U1/simple model/B ==
  data: f input; m input; R_dot input; B output; W input
function B  = fcn(f, m, R_dot, W)
B = [(1/m)*R_dot*f*W; zeros(3,1)];
end

== matlab function simple_controll/control/U1/simple model/J ==
  data: Th input; J output; f output
function [J, f] = fnc(Th)
J = J_fcn(Th(1), Th(2), Th(3), Th(4));
f = J(1:3, 1:4);
end

== matlab function simple_controll/control/U1/simple model/Jr ==
  data: R_BI input; Jr output; m input; I_B input

function Jr = fcn(R_BI, m, I_B)
Jr = [(1/m)*R_BI zeros(3);
      zeros(3) I_B^(-1)];
end

== matlab function simple_controll/control/U1/simple model/dJ_w ==
  data: W input; Th input; dJ_w output
function dJ_w = fcn(W, Th)
    dJ_w = dJ_w_fcn(Th(1), Th(2), Th(3), Th(4), W(1), W(2), W(3), W(4));
end

== matlab function simple_controll/control/new control1/A B/A, Apinv  ==
  data: J input; Jr input; A output; Apinv output
function [A,Apinv]= fcn(J, Jr)
A = Jr * J;
Apinv = pinv(A);
end

== matlab function simple_controll/control/new control1/A B/J ==
  data: Th input; J output
function J  = fnc(Th)
J = J_fcn(Th(1), Th(2), Th(3), Th(4));
end

== matlab function simple_controll/control/new control1/A B/Jr ==
  data: R_BI input; Jr output; m input; I_B input

function Jr = fcn(R_BI, m, I_B)
Jr = [(1/m)*R_BI zeros(3);
      zeros(3) I_B^(-1)];
end

== matlab function simple_controll/control/new control1/A B/U(W) ==
  data: g input; pinvA input; W output size=4; error input
function W = fcn(g, pinvA, error)
W = pinvA*(error - [g;0;0;0]);
end

== matlab function simple_controll/control/new control1/Th ==
  data: Th output size=4; err input; R_BI input
function Th = fnc(err, R_BI)

rm = err(1:3);

R_IB = R_BI';
rm = R_IB*rm;
cx = rm(1)/(rm(3)+1*sign(rm(3)));
cy = rm(2)/(rm(3)+1*sign(rm(3)));

Ths = resolve_th(cx, cy);
ThA = Ths(1, :)';
ThB = Ths(2, :)';

if max(abs(ThA)) < max(abs(ThB))
    Th = ThA;
else
    Th = ThB;
end
for i = 1:4
    Th(i) = sign(Th(i))*min(abs(Th(i)), pi/3);
end


end

== matlab function simple_controll/control/new control1/error/e_R ==
  data: R_d input; R_r input; e_R output size=3
function e_R = e_r(R_d, R_r)
Me_R = R_r'*R_d - R_d'*R_r;
e_R = 0.5*[-Me_R(2,3); Me_R(1,3); -Me_R(1,2)];
end

== matlab function simple_controll/control/new control1/error/e_r ==
  data: r input; d input; e output size=3; lim input
function e = e_r(r, d, lim)
e = d - r;
n = norm(e);
if n < lim
    return;
end
e = lim*e/n;
end

== matlab function simple_controll/control/new control1/error/e_rdot ==
  data: r input; d input; e output size=3; lim input
function e = e_r(r, d, lim)
e = d - r;
n = norm(e);
if n < lim
    return;
end
e = lim*e/n;
end

== matlab function simple_controll/control/new control1/error/e_w ==
  data: r input; d input; e output size=3; lim input
function e = e_r(r, d, lim)
e = d - r;
n = norm(e);
if n < lim
    return;
end
e = lim*e/n;
end

== matlab function simple_controll/control/new control1/error/error1 ==
  data: r_err input; rdot_err input; error output; r2dot_d input; e_R input; w_err input; wdot_d input
function error = x_e(r_err, rdot_err, r2dot_d, e_R, w_err, wdot_d)
   
K1 = 3*[1,0,0;
      0,1,0;
      0,0,1]*80;

K0 =  3*[1,0,0;
       0,1,0;
       0,0,1]*100;
   
e_x =  r2dot_d + K1*(rdot_err)+ K0*(r_err);

C1 =   [1,0,0;
        0,1,0;
        0,0,1]*200;

C0 =   [1,0,0;
        0,1,0;
        0,0,1.6]*500;
          
e_r = wdot_d + C1*(w_err) + C0*(e_R);
error = [e_x; e_r];
end

== matlab function simple_controll/control/new control1/error/omegad ==
  data: omega output; RBIdot input; RBI input
function omega  = fcn(RBIdot, RBI)

R = RBI'*RBIdot;
omega = [-R(2,3); R(1,3); -R(1,2)];

== matlab function simple_controll/control/new control1/q2R ==
  data: qBI input; R output
function R = q2R(qBI)
R = quat2matrix(qBI);
end
